simulink model "encoderModel"  (R2015a)
settings: Solver=ode45  StartTime=0.0  StopTime=20  RelTol=1e-3
settings Model: Creator=dell  LastModifiedBy=dell

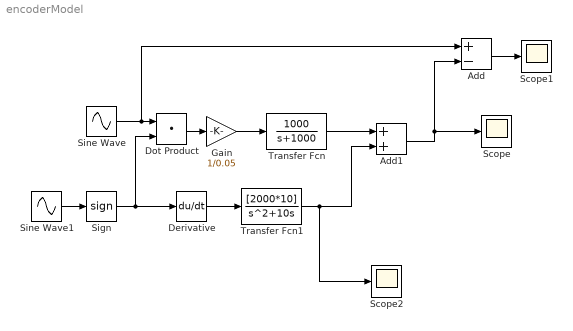
== system encoderModel ==
  Add : Sum  Inputs=+-
  Add1 : Sum
  Derivative : Derivative
  Dot Product : DotProduct  InputSameDT=on  OutDataTypeStr=Inherit: Inherit via internal rule
  Gain : Gain  Gain=1/0.05
  Scope : Scope
  Scope1 : Scope
  Scope2 : Scope
      settings: SaveName=ScopeData2
  Sign : Signum
  Sine Wave : Sin  Frequency=2*pi  SampleTime=0
  Sine Wave1 : Sin  Frequency=2*pi*0.1  SampleTime=0
  Transfer Fcn : TransferFcn  Numerator=[1000]  Denominator=[1 1000]
  Transfer Fcn1 : TransferFcn  Numerator=[2000*10]  Denominator=[1 10 0]
  wires:
  Gain/1 -> Transfer Fcn/1
  Sine Wave/1 -> Add/1, Dot Product/1
  Dot Product/1 -> Gain/1
  Sign/1 -> Derivative/1, Dot Product/2
  Sine Wave1/1 -> Sign/1
  Add/1 -> Scope1/1
  Derivative/1 -> Transfer Fcn1/1
  Transfer Fcn/1 -> Add1/1
  Transfer Fcn1/1 -> Scope2/1, Add1/2
  Add1/1 -> Scope/1, Add/2
